simulink model "SHUNT_ACTIVE_FILTER"  (R2025b)
settings: Solver=ode23t  StartTime=0.0  StopTime=0.25  RelTol=1e-3
libraries: spsThreePhaseVIMeasurementLib x3, spsabctodq0Lib x2, spsUniversalBridgeLib x2, spsDCVoltageSourceLib x1, spsPLL3phLib x1, spsPowerdq0InstantaneousLib x1, eeGeneralControl x1, spsdq0toabcLib x1, spsSeriesRLCBranchLib x1, spsThreePhaseSeriesRLCBranchLib x1, spsThreePhaseSourceLib x1, sps_lib x1
settings Model: Creator=Asus  LastModifiedBy=Asus
settings DataIOCC: ReturnWorkspaceOutputs=off

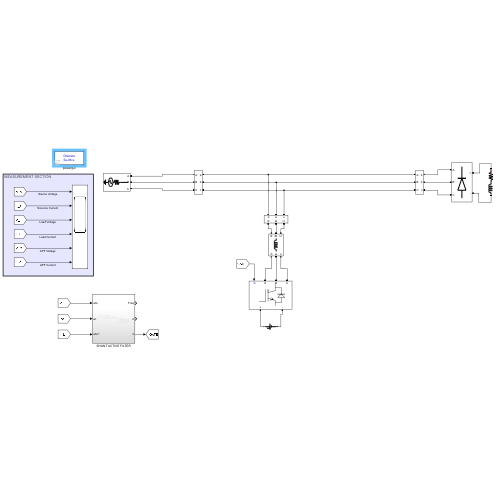
[thumbnail: Simulink's stored preview of the top-level diagram]
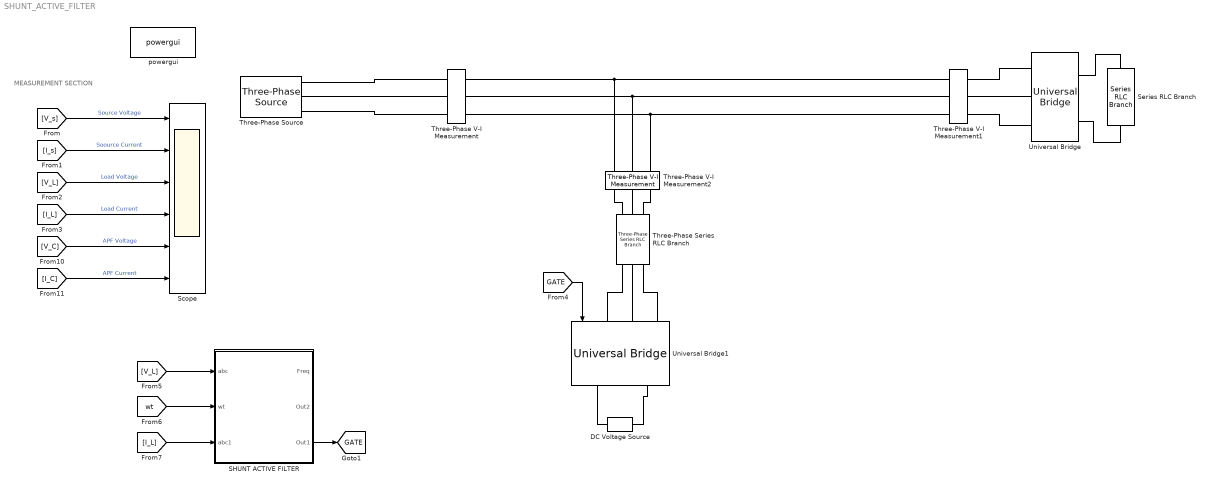
== system SHUNT_ACTIVE_FILTER ==
  note: MEASUREMENT SECTION
  DC Voltage Source : spsDCVoltageSourceLib/DC Voltage Source  Amplitude=700  Measurements=None
  SHUNT ACTIVE FILTER : Subsystem
  Scope : Scope  NumInputPorts=6
      settings: ActiveDisplayYMinimum=-269.95651518455907  ActiveDisplayYMaximum=496.94683357745259
  Series RLC Branch : spsSeriesRLCBranchLib/Series RLC Branch  LConnTagsString=__new0  RConnTagsString=__new0  BranchType=RL  Resistance=10  Inductance=2e-3  SetiL0=off  InitialCurrent=0  Capacitance=1e-6  Setx0=off  InitialVoltage=0  Measurements=None
  Three-Phase Series RLC Branch : spsThreePhaseSeriesRLCBranchLib/Three-Phase Series RLC Branch  LConnTagsString=A|B|C  RConnTagsString=A|B|C  BranchType=L  Resistance=1  Inductance=2e-3  Capacitance=1e-6  Measurements=None
  Three-Phase V-I Measurement : spsThreePhaseVIMeasurementLib/Three-Phase V-I Measurement  VoltageMeasurement=phase-to-ground  SetLabelV=on  LabelV=V_s  Vpu=off  VpuLL=off  CurrentMeasurement=yes  SetLabelI=on  LabelI=I_s  Ipu=off  Pbase=100e6  Vbase=500e3  OutputType=Complex  PhasorSimulation=off  PSBequivalent=0
  Three-Phase V-I Measurement1 : spsThreePhaseVIMeasurementLib/Three-Phase V-I Measurement  VoltageMeasurement=phase-to-ground  SetLabelV=on  LabelV=V_L  Vpu=off  VpuLL=off  CurrentMeasurement=yes  SetLabelI=on  LabelI=I_L  Ipu=off  Pbase=100e6  Vbase=500e3  OutputType=Complex  PhasorSimulation=off  PSBequivalent=0
  Three-Phase V-I Measurement2 : spsThreePhaseVIMeasurementLib/Three-Phase V-I Measurement  VoltageMeasurement=phase-to-ground  SetLabelV=on  LabelV=V_C  Vpu=off  VpuLL=off  CurrentMeasurement=yes  SetLabelI=on  LabelI=I_C  Ipu=off  Pbase=100e6  Vbase=500e3  OutputType=Complex  PhasorSimulation=off  PSBequivalent=0
  Three-Phase Source : spsThreePhaseSourceLib/Three-Phase Source  InternalConnection=Yg  VoltagePhases=off  Voltage=400  PhaseAngle=0  Voltage_phases=[25e3 25e3 25e3]/sqrt(3)  PhaseAngles_phases=[0 -120 +120]  Frequency=50  NonIdealSource=on  SpecifyImpedance=off  Resistance=0.9  Inductance=0  ShortCircuitLevel=100e6  BaseVoltage=400  XRratio=7  BusType=swing  Pref=10e3  Qref=0  Prefabc=[10e3, 10e3, 10e3]  Qrefabc=[0, 0, 0]  Qmin=-inf  Qmax=inf
  Universal Bridge : spsUniversalBridgeLib/Universal Bridge  Arms=3  SnubberResistance=1e5  SnubberCapacitance=inf  Device=Diodes  Ron=1e-3  Lon=0  ForwardVoltages="[  0  0  ]"  ForwardVoltage=0  GTOparameters=[ 10e-6 , 20e-6 ]  IGBTparameters=[ 1e-6 , 2e-6 ]  Measurements=None  Measurements_2=None  converterType=Rectifier
  Universal Bridge1 : spsUniversalBridgeLib/Universal Bridge  Arms=3  SnubberResistance=1e5  SnubberCapacitance=inf  Device=IGBT / Diodes  Ron=1e-3  Lon=0  ForwardVoltages="[  0  0  ]"  ForwardVoltage=0  GTOparameters=[ 10e-6 , 20e-6 ]  IGBTparameters=[ 1e-6 , 2e-6 ]  Measurements=None  Measurements_2=None  converterType=Rectifier
  powergui : sps_lib/powergui  Priority=1  SimulationMode=Discrete  SampleTime=5e-6  frequency=60  Iterations=50  frequencyindice=0  Pbase=100e6  ErrMax=1e-4  UnitsV=kV  UnitsW=MW  buscounter=0  FunctionMessages=off  echomessages=off  EnableUseOfTLC=off  CurrentSourceSwitches=off  DisableSnubberDevices=off  DisableRonSwitches=off  DisableVfSwitches=off  DisplayEquations=off  AutomaticDiscreteSolvers=off  SolverType=Tustin/Backward Euler (TBE)  Interpol=off  ExternalGateDelay=off  methode=off  Ts=100  x0status=blocks  SPID=on  SwTol=0  HookPort=off  NonlinearTolerance=1e-4  nMaxIteration=100  ContinueOnMaxIteration=off  RestoreLinks=warning  ResistiveCurrentMeasurement=off  Frange=[0:2:500]  Ylog=off  Xlog=on  ShowGrid=off  save=off  variable=ZData  structure=0  ZoomFFT=off  StartTime=0.0  cycles=1  DisplayStyle=1  fundamental=60  FreqAxis=off  MaxFrequency=1000  frequencyindicesteady=1  RmsSteady=1  display=off
  tag scope: GATE=global
  wires:
  [V_s] -> Scope/1  "Source Voltage"
  [I_s] -> Scope/2  "Soource Current"
  [V_L] -> Scope/3  "Load Voltage"
  [GATE] -> Universal Bridge1/1
  [I_L] -> Scope/4  "Load Current"
  [V_C] -> Scope/5  "APF Voltage"
  [I_C] -> Scope/6  "APF Current"
  [V_L] -> SHUNT ACTIVE FILTER/1(abc)
  [wt] -> SHUNT ACTIVE FILTER/2(wt)
  [I_L] -> SHUNT ACTIVE FILTER/3(abc1)
  SHUNT ACTIVE FILTER/3(Out1) -> [GATE]
  connections:
  Universal Bridge/RConn1 -- Series RLC Branch/LConn1
  Universal Bridge/RConn2 -- Series RLC Branch/RConn1
  Three-Phase V-I Measurement2/RConn1 -- Three-Phase V-I Measurement/RConn1 -- Three-Phase V-I Measurement1/LConn1
  Three-Phase V-I Measurement1/LConn2 -- Three-Phase V-I Measurement2/RConn2 -- Three-Phase V-I Measurement/RConn2
  Three-Phase V-I Measurement1/LConn3 -- Three-Phase V-I Measurement2/RConn3 -- Three-Phase V-I Measurement/RConn3
  Three-Phase V-I Measurement1/RConn2 -- Universal Bridge/LConn2
  Three-Phase V-I Measurement1/RConn1 -- Universal Bridge/LConn1
  Three-Phase V-I Measurement1/RConn3 -- Universal Bridge/LConn3
  DC Voltage Source/RConn1 -- Universal Bridge1/RConn1
  Three-Phase Series RLC Branch/RConn2 -- Universal Bridge1/LConn2
  Three-Phase Series RLC Branch/RConn3 -- Universal Bridge1/LConn3
  Three-Phase Series RLC Branch/RConn1 -- Universal Bridge1/LConn1
  Three-Phase V-I Measurement2/LConn2 -- Three-Phase Series RLC Branch/LConn2
  Three-Phase Series RLC Branch/LConn3 -- Three-Phase V-I Measurement2/LConn3
  Three-Phase Series RLC Branch/LConn1 -- Three-Phase V-I Measurement2/LConn1
  DC Voltage Source/LConn1 -- Universal Bridge1/RConn2
  Three-Phase Source/RConn2 -- Three-Phase V-I Measurement/LConn2
  Three-Phase Source/RConn3 -- Three-Phase V-I Measurement/LConn3
  Three-Phase Source/RConn1 -- Three-Phase V-I Measurement/LConn1

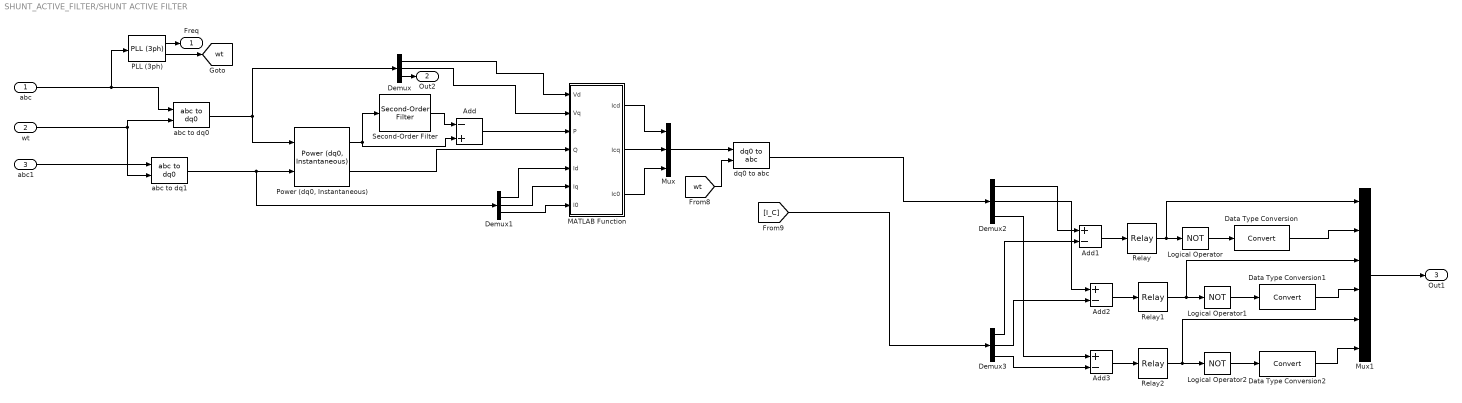
== system SHUNT_ACTIVE_FILTER/SHUNT ACTIVE FILTER ==
  abc : Inport
  wt : Inport  Port=2
  abc1 : Inport  Port=3
  Add : Sum  Inputs=-+
  Add1 : Sum  Inputs=+-
  Add2 : Sum  Inputs=+-
  Add3 : Sum  Inputs=+-
  Data Type Conversion : DataTypeConversion  SaturateOnIntegerOverflow=off  RndMeth=Floor
  Data Type Conversion1 : DataTypeConversion  SaturateOnIntegerOverflow=off  RndMeth=Floor
  Data Type Conversion2 : DataTypeConversion  SaturateOnIntegerOverflow=off  RndMeth=Floor
  Demux{,1..3} (4 alike) : Demux  Outputs=3
  Logical Operator : Logic  Operator=NOT  AllPortsSameDT=off  OutDataTypeStr=boolean
  Logical Operator1 : Logic  Operator=NOT  AllPortsSameDT=off  OutDataTypeStr=boolean
  Logical Operator2 : Logic  Operator=NOT  AllPortsSameDT=off  OutDataTypeStr=boolean
  MATLAB Function : MATLAB Function  TreatAsAtomicUnit=on
  Mux : Mux  Inputs=3
  Mux1 : Mux  Inputs=6
  PLL (3ph) : spsPLL3phLib/PLL (3ph)  Fmin=45  Par_Init=[0, 50]  ParK=[180, 3200, 1]  TcD=1e-4  MaxRateChangeFreq=12  FilterCutOffFreq=5  Ts=0  AGC=on
  "Power (dq0, Instantaneous)" : spsPowerdq0InstantaneousLib/Power (dq0, Instantaneous)
      settings: LibrarySourceBlock=|
      | sps_lib/Sensors and Measurements/Power
      | (dq0, Instantaneous)
  Relay : Relay  OnSwitchValue=0.01  OffSwitchValue=0.01
  Relay1 : Relay  OnSwitchValue=0.01  OffSwitchValue=0.01
  Relay2 : Relay  OnSwitchValue=0.01  OffSwitchValue=0.01
  Second-Order Filter : eeGeneralControl/Second-Order Filter  FilterType=Low-pass  fn=10  Zeta=0.707  Ts=-1  A0=0  Ph0=0  f0=0  b0=0
      settings: LibrarySourceBlock=ee_sl_lib/General Control/Second-Order Filter
  abc to dq0 : spsabctodq0Lib/abc to dq0  Alignment=90 degrees behind phase A axis
  abc to dq1 : spsabctodq0Lib/abc to dq0  Alignment=90 degrees behind phase A axis
  dq0 to abc : spsdq0toabcLib/dq0 to abc  Alignment=90 degrees behind phase A axis
  Freq : Outport
  Out2 : Outport  Port=2
  Out1 : Outport  Port=3
  tag scope: wt=global
  wires:
  abc/1 -> abc to dq0/1, PLL (3ph)/1
  MATLAB Function/2(Icq) -> Mux/2
  Mux/1 -> dq0 to abc/1
  abc to dq1/1 -> Demux1/1, "Power (dq0, Instantaneous)"/2
  Second-Order Filter/1 -> Add/1
  Demux/2 -> MATLAB Function/2(Vq)
  Demux/1 -> MATLAB Function/1(Vd)
  abc1/1 -> abc to dq1/1
  MATLAB Function/3(Ic0) -> Mux/3
  "Power (dq0, Instantaneous)"/2 -> MATLAB Function/4(Q)
  Demux1/3 -> MATLAB Function/7(I0)
  PLL (3ph)/2 -> [wt]
  "Power (dq0, Instantaneous)"/1 -> Second-Order Filter/1, Add/2
  Demux1/2 -> MATLAB Function/6(Iq)
  wt/1 -> abc to dq0/2, abc to dq1/2
  [wt] -> dq0 to abc/2
  Demux1/1 -> MATLAB Function/5(Id)
  MATLAB Function/1(Icd) -> Mux/1
  Add/1 -> MATLAB Function/3(P)
  abc to dq0/1 -> Demux/1, "Power (dq0, Instantaneous)"/1
  Demux/3 -> Out2/1
  PLL (3ph)/1 -> Freq/1
  Data Type Conversion1/1 -> Mux1/4
  Data Type Conversion/1 -> Mux1/2
  Demux2/3 -> Add3/1
  Demux3/1 -> Add1/2
  Data Type Conversion2/1 -> Mux1/6
  Add3/1 -> Relay2/1
  Mux1/1 -> Out1/1
  Logical Operator/1 -> Data Type Conversion/1
  Demux3/2 -> Add2/2
  Add1/1 -> Relay/1
  Logical Operator1/1 -> Data Type Conversion1/1
  Demux2/1 -> Add1/1
  Logical Operator2/1 -> Data Type Conversion2/1
  Add2/1 -> Relay1/1
  Relay2/1 -> Mux1/5, Logical Operator2/1
  Relay/1 -> Mux1/1, Logical Operator/1
  Demux2/2 -> Add2/1
  Relay1/1 -> Mux1/3, Logical Operator1/1
  Demux3/3 -> Add3/2
  dq0 to abc/1 -> Demux2/1
  [I_C] -> Demux3/1

== matlab function SHUNT_ACTIVE_FILTER/SHUNT ACTIVE FILTER/MATLAB Function ==
  data: Vd input; Icd output; Vq input; P input; Q input; Id input; Iq input; I0 input; Icq output; Ic0 output
function [Icd, Icq, Ic0] = fcn(Vd, Vq, P, Q, Id, Iq, I0)

Icd=(2/3)*(1/(Vd^2+Vq^2))*(Vd*P+Vq*Q);
Icq=(2/3)*(1/(Vd^2+Vq^2))*(Vq*P-Vd*Q);
Ic0=I0
